simulink model "prbs_4bits"  (Simulink 7.9)
settings: Solver=FixedStepDiscrete  StartTime=0.0  StopTime=15  FixedStep=1  RelTol=1e-3
undefined symbols (not defined in the file): TS_PRBS
settings Model: Creator=bailly  LastModifiedBy=matias
settings OptimizationCC: InitFltsAndDblsToZero=on
settings DebuggingCC: SaveWithParameterizedLinksMsg=none  FcnCallInpInsideContextMsg=Use local settings  StrictBusMsg=Warning
settings GRTTargetCC: TargetFcnLib=ansi_tfl_tmw.mat  CombineOutputUpdateFcns=off  GRTInterface=on

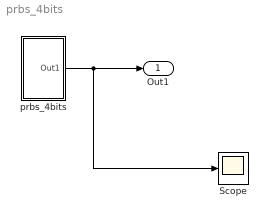
== system prbs_4bits ==
  Scope : Scope
  prbs_4bits : Subsystem
  Out1 : Outport
  wires:
  prbs_4bits/1(Out1) -> Out1/1, Scope/1

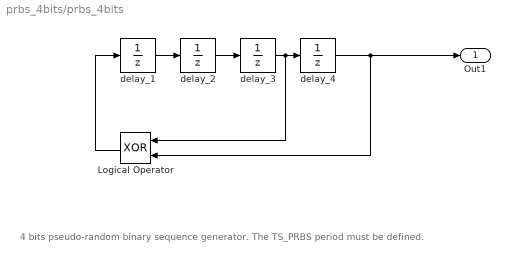
== system prbs_4bits/prbs_4bits ==
  note: 4 bits pseudo-random binary sequence generator.
      | The TS_PRBS period must be defined.
  Logical Operator : Logic  Operator=XOR  AllPortsSameDT=off  OutDataTypeStr=boolean
  delay_1 : UnitDelay  X0=1  SampleTime=TS_PRBS
  delay_2 : UnitDelay  X0=1  SampleTime=-1
  delay_3 : UnitDelay  X0=1  SampleTime=-1
  delay_4 : UnitDelay  X0=1  SampleTime=-1
  Out1 : Outport
  wires:
  delay_2/1 -> delay_3/1
  delay_3/1 -> delay_4/1, Logical Operator/1
  delay_4/1 -> Logical Operator/2, Out1/1
  delay_1/1 -> delay_2/1
  Logical Operator/1 -> delay_1/1
